simulink model "V605_motorModel"  (R2024a)
settings: Solver=VariableStepAuto  StartTime=0.0  StopTime=10.0  RelTol=1e-3
model workspace (MAT data in the model file):
  Sig = Simulink.Signal
  Sig.DataType = 'auto'
  Sig.Dimensions = -1
  Sig.DimensionsMode = 'auto'
  Sig.Complexity = 'auto'
  Sig.SampleTime = -1
  Sig.SamplingMode = 'auto'
settings Model: Creator=Tristan  LastModifiedBy=Tristan

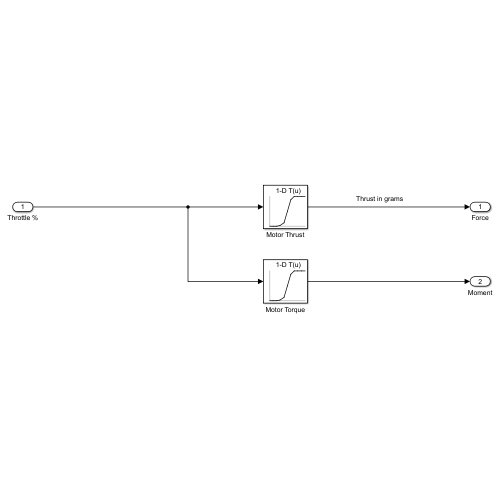
[thumbnail: Simulink's stored preview of the top-level diagram]
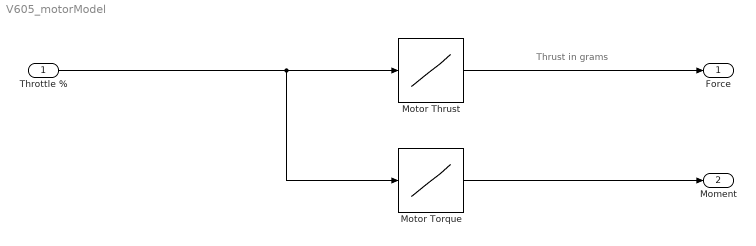
== system V605_motorModel ==
  note: Thrust in grams
  Throttle % : Inport
  Motor Thrust : Lookup_n-D  NumberOfTableDimensions=1  BreakpointsForDimension1=[-5:5]  Table=tanh([-5:5])  InternalRulePriority=Speed  RndMeth=Simplest
  Motor Torque : Lookup_n-D  NumberOfTableDimensions=1  BreakpointsForDimension1=[-5:5]  Table=tanh([-5:5])  InternalRulePriority=Speed  RndMeth=Simplest
  Force : Outport
  Moment : Outport  Port=2
  wires:
  Motor Thrust/1 -> Force/1
  Throttle %/1 -> Motor Torque/1, Motor Thrust/1
  Motor Torque/1 -> Moment/1
